simulink model "SAE"  (R2018a)
settings: Solver=VariableStepAuto  StartTime=0.0  StopTime=stoptime  RelTol=1e-3
values from neighbouring files (symbols this model uses):
  A = [Xu Xw -aa0*U0 -g*cos(tt0) ... (first row only)    [Model.m]
  B = [Xde Xdt ... (first row only)    [Model.m]
  C = eye(4)    [Model.m]
  D = zeros(4,2)    [Model.m]
  kq = 2.2890    (= 2.289)    [Model.m]
  ku = 0.0654    [Model.m]
  stoptime = 500    [Model.m]
settings Model: Creator=beapedroso  LastModifiedBy=tfesc

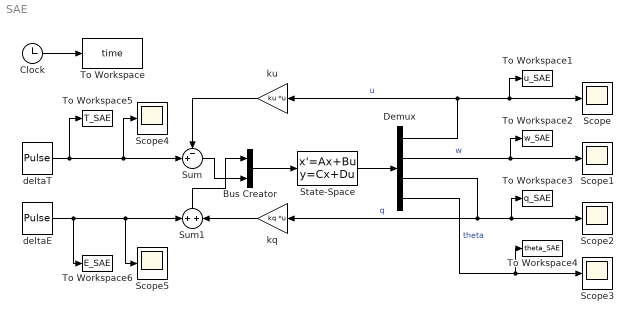
== system SAE ==
  Bus Creator : BusCreator  Inputs=2
  Clock : Clock
  Demux : Demux
  Scope{,1..5} (6 alike) : Scope
  State-Space : StateSpace  A=A  B=B  C=C  D=D  InitialCondition=0
  Sum : Sum  Inputs=-+|
  Sum1 : Sum  Inputs=+|+
  To Workspace : ToWorkspace  VariableName=time  SampleTime=-1
  To Workspace1 : ToWorkspace  VariableName=u_SAE  SampleTime=-1
  To Workspace2 : ToWorkspace  VariableName=w_SAE  SampleTime=-1
  To Workspace3 : ToWorkspace  VariableName=q_SAE  SampleTime=-1
  To Workspace4 : ToWorkspace  VariableName=theta_SAE  SampleTime=-1
  To Workspace5 : ToWorkspace  VariableName=T_SAE  SaveFormat=Structure  SampleTime=-1
  To Workspace6 : ToWorkspace  VariableName=E_SAE  SampleTime=-1
  "deltaE " : DiscretePulseGenerator  PulseType=Time based  Amplitude=3*3.14/180  Period=stoptime  PulseWidth=15  PhaseDelay=300
  deltaT : DiscretePulseGenerator  PulseType=Time based  Amplitude=0.1  Period=stoptime  PulseWidth=10  PhaseDelay=10
  kq : Gain  Gain=kq  Multiplication=Matrix(K*u)
  ku : Gain  Gain=ku  Multiplication=Matrix(K*u)
  wires:
  Demux/2 -> To Workspace2/1, Scope1/1  "w"
  Demux/4 -> To Workspace4/1, Scope3/1  "theta"
  State-Space/1 -> Demux/1
  Demux/1 -> ku/1, To Workspace1/1, Scope/1  "u"
  Demux/3 -> To Workspace3/1, Scope2/1, kq/1  "q"
  Clock/1 -> To Workspace/1
  ku/1 -> Sum/1
  deltaT/1 -> To Workspace5/1, Scope4/1, Sum/2
  Bus Creator/1 -> State-Space/1
  kq/1 -> Sum1/2
  "deltaE "/1 -> To Workspace6/1, Scope5/1, Sum1/1
  Sum1/1 -> Bus Creator/1
  Sum/1 -> Bus Creator/2
